simulink model "r2dbe_top"  (R2012b)
settings: Solver=VariableStepDiscrete  SolverMode=SingleTasking  StartTime=0.0  StopTime=10000  RelTol=1e-3
undefined symbols (not defined in the file or in its folder): r2dbe_vdif_lib, sfp, vdif
libraries: xbsIndex_r4 x2792, dspsigops x32, casper_library_delays x29, casper_library_sources x16, casper_library_misc x12, r2dbe_adc_lib x5, xps_library x4, simulink x2
(part 1 of 28)
settings Model: Creator=rprimian  LastModifiedBy=ayoung
settings DataIOCC: SignalLoggingSaveFormat=ModelDataLogs
settings OptimizationCC: InlineParams=on
settings DebuggingCC: SolverPrmCheckMsg=none  FcnCallInpInsideContextMsg=UseLocalSettings  StrictBusMsg=Warning
settings GRTTargetCC: CombineOutputUpdateFcns=off  GRTInterface=on

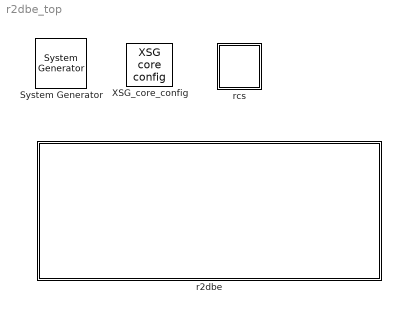
== system r2dbe_top ==
  " System Generator" : xbsIndex_r4/ System Generator  Tag=genX  xilinxfamily=virtex6  part=xc6vsx475t  speed=-1  package=ff1759  synthesis_tool=XST  clock_wrapper=Clock Enables  directory=./r2dbe_top/sysgen  proj_type=Project Navigator  Synth_file=XST Defaults  Impl_file=ISE Defaults  testbench=off  simulink_period=1  sysclk_period=3.9062  dcm_input_clock_period=100  incr_netlist=off  trim_vbits=Everywhere in SubSystem  dbl_ovrd=According to Block Masks  core_generation=According to Block Masks  run_coregen=off  deprecated_control=off  eval_field=0  block_type=sysgen
      settings: block_version=11.4
  XSG_core_config : xps_library/XSG core config  Tag=xps:xsg  hw_sys=ROACH2:sx475t  clk_src=adc0_clk  ROACH_clk_src=dac1_clk  ROACH2_clk_src=adc0_clk  MKDIG_clk_src=sys_clk  clk_rate=256.0  sample_period=1  synthesis_tool=XST
  r2dbe : Subsystem
  rcs : Subsystem  AncestorBlock=casper_library_misc/rcs  mask(rcs){app_src=timestamp, lib_src=git, user_val=2704}
      mask prompts: app_src "Application revision info to capture"; lib_src "CASPER libraries revision info to capture"; user_val "User specified value"
      mask help:
      | Embeds revision control information for the user design and libraries.
      | On failure to locate specified revision information, falls back to
      | timestamps (current time for libraries).
      | A user specified value is also stored.
      mask init:
      | rcs_init(gcb, ...
      |     'app_src', app_src, ...
      |     'lib_src', lib_src);
      mask TypeOptions app_src: timestamp | git | svn
      mask TypeOptions lib_src: timestamp | git | svn

== system r2dbe_top/r2dbe ==
  1PPS : DiscretePulseGenerator  Period=10
  IF0 Band : simulink/Sources/Band-Limited White Noise  Cov=[0.1]  Ts=1  seed=[23341]
  IF1 Band : simulink/Sources/Band-Limited White Noise  Cov=[0.1]  Ts=1  seed=[23341]
  data_mux_0 : Subsystem  mask(r2dbe_data_mux){mux_latency=1, pipeline_delay=1}
      mask prompts: mux_latency "Mux latency:"; pipeline_delay "Output pipeline delay:"
      mask help: Sub-system for mux parameters of the R2DBE.
      mask Display:
      | plot([0 45 45 0 0 ],[0 14.8571 89.1429 104 0 ]);
      | 
      | color('black');port_label('input',1,'sync_in');
      | color('black');port_label('input',2,'adc');
      | color('black');port_label('input',3,'noise');
      | color('black');port_label('input',4,'tone');
      | 
      | color('black');port_label('output',1,'sync');
      | color('black');port_label('output',2,'out');
      | 
      | color('black');disp('\bf{}','texmode','on');
  data_mux_1 : Subsystem  mask(r2dbe_data_mux){mux_latency=1, pipeline_delay=1}
      mask prompts: mux_latency "Mux latency:"; pipeline_delay "Output pipeline delay:"
      mask help: Sub-system for mux parameters of the R2DBE.
      mask Display:
      | plot([0 45 45 0 0 ],[0 14.8571 89.1429 104 0 ]);
      | 
      | color('black');port_label('input',1,'sync_in');
      | color('black');port_label('input',2,'adc');
      | color('black');port_label('input',3,'noise');
      | color('black');port_label('input',4,'tone');
      | 
      | color('black');port_label('output',1,'sync');
      | color('black');port_label('output',2,'out');
      | 
      | color('black');disp('\bf{}','texmode','on');
  delay_0 : Subsystem  mask(r2dbe_delay){max_delay=256, bram_latency=4, pipeline_delay=3}
      mask prompts: max_delay "Max Delay (samples):"; bram_latency "BRAM Latency:"; pipeline_delay "Output pipeline delay:"
      mask help: Sub-system for delay parameters of the R2DBE.
  delay_1 : Subsystem  mask(r2dbe_delay){max_delay=256, bram_latency=4, pipeline_delay=3}
      mask prompts: max_delay "Max Delay (samples):"; bram_latency "BRAM Latency:"; pipeline_delay "Output pipeline delay:"
      mask help: Sub-system for delay parameters of the R2DBE.
  noise_gen_0 : Subsystem  AncestorBlock=r2dbe_adc_lib/noise_gen  mask(r2dbe_noise_gen){}
      mask help: Sub-system for noise generation of the R2DBE.
  noise_gen_1 : Subsystem  AncestorBlock=r2dbe_adc_lib/noise_gen  mask(r2dbe_noise_gen){}
      mask help: Sub-system for noise generation of the R2DBE.
  onepps : Subsystem  AncestorBlock=r2dbe_adc_lib/onepps  mask(r2dbe_onepps){clk_rate=4096 / 16}
      mask prompts: clk_rate "FPGA clock rate (MHz):"
      mask help: Sub-system for 1pps parameters of the R2DBE.
  quantize_0 : r2dbe_adc_lib/quantize  mult_delay=3  add_delay=2  convert_delay=1  pipeline_delay=1  io_delay=3
      link override thresh/io_delay: latency=0  reg_retiming=on
      link override thresh/r2dbe_top_r2dbe_quantize_0_thresh_user_data_out: arith_type=Unsigned  n_bits=32  bin_pt=0  period=1
      link override thresh/reint1: force_arith_type=on  arith_type=Unsigned  force_bin_pt=on  bin_pt=0
      link override thresh/slice_gain: nbits=32  boolean_output=off  mode=Lower Bit Location + Width  bit0=0
  quantize_1 : r2dbe_adc_lib/quantize  mult_delay=3  add_delay=2  convert_delay=1  pipeline_delay=1  io_delay=3
      link override thresh/io_delay: latency=0  reg_retiming=on
      link override thresh/r2dbe_top_r2dbe_quantize_1_thresh_user_data_out: arith_type=Unsigned  n_bits=32  bin_pt=0  period=1
      link override thresh/reint1: force_arith_type=on  arith_type=Unsigned  force_bin_pt=on  bin_pt=0
      link override thresh/slice_gain: nbits=32  boolean_output=off  mode=Lower Bit Location + Width  bit0=0
  snap_2bit_0 : Subsystem  mask(r2dbe_snap){nsamples=14, data_width=32, io_delay=6}
      mask prompts: nsamples "Number of samples (2^?):"; data_width "Data width (bits):"; io_delay "I/O delay:"
      mask help: Sub-system for snapshot parameters of the R2DBE.
      mask init:
      | set_param([gcb, '/data'], 'data_width', data_width);
      mask TypeOptions data_width: 8 | 16 | 32 | 64 | 128
  snap_2bit_1 : Subsystem  mask(r2dbe_snap){nsamples=14, data_width=32, io_delay=6}
      mask prompts: nsamples "Number of samples (2^?):"; data_width "Data width (bits):"; io_delay "I/O delay:"
      mask help: Sub-system for snapshot parameters of the R2DBE.
      mask init:
      | set_param([gcb, '/data'], 'data_width', data_width);
      mask TypeOptions data_width: 8 | 16 | 32 | 64 | 128
  snap_8bit_0 : Subsystem  mask(r2dbe_snap){nsamples=14, data_width=128, io_delay=6}
      mask prompts: nsamples "Number of samples (2^?):"; data_width "Data width (bits):"; io_delay "I/O delay:"
      mask help: Sub-system for snapshot parameters of the R2DBE.
      mask init:
      | set_param([gcb, '/data'], 'data_width', data_width);
      mask TypeOptions data_width: 8 | 16 | 32 | 64 | 128
  snap_8bit_1 : Subsystem  mask(r2dbe_snap){nsamples=14, data_width=128, io_delay=6}
      mask prompts: nsamples "Number of samples (2^?):"; data_width "Data width (bits):"; io_delay "I/O delay:"
      mask help: Sub-system for snapshot parameters of the R2DBE.
      mask init:
      | set_param([gcb, '/data'], 'data_width', data_width);
      mask TypeOptions data_width: 8 | 16 | 32 | 64 | 128
  tengbe_0 : Subsystem  mask(r2dbe_tengbe){slot=0, port=0}
      mask prompts: slot "Card slot:"
      mask help: Sub-system for 10 GbE parameters of the R2DBE.
      mask init:
      | set_param([gcb, '/core'], 'slot', slot);
      | set_param([gcb, '/core'], 'port_r2_sfpp', port);
      mask TypeOptions slot: 0 | 1
      mask TypeOptions port: 0 | 1 | 2 | 3
  tengbe_1 : Subsystem  mask(r2dbe_tengbe){slot=0, port=1}
      mask prompts: slot "Card slot:"
      mask help: Sub-system for 10 GbE parameters of the R2DBE.
      mask init:
      | set_param([gcb, '/core'], 'slot', slot);
      | set_param([gcb, '/core'], 'port_r2_sfpp', port);
      mask TypeOptions slot: 0 | 1
      mask TypeOptions port: 0 | 1 | 2 | 3
  tone_gen_1 : Subsystem  mask(r2dbe_tone_gen){}
      mask help: Sub-system for tone generation of the R2DBE.
  tone_gen_2 : Subsystem  mask(r2dbe_tone_gen){}
      mask help: Sub-system for tone generation of the R2DBE.
  vdif_0 : Subsystem  AncestorBlock=r2dbe_vdif_lib/vdif  mask(r2dbe_vdif){}
      mask help: Sub-system for VDIF parameters of the R2DBE.
  vdif_1 : Subsystem  AncestorBlock=r2dbe_vdif_lib/vdif  mask(r2dbe_vdif){}
      mask help: Sub-system for VDIF parameters of the R2DBE.
  zdok_0 : Subsystem  mask(r2dbe_zdok){zdok=ZDOK 0, nyquist_bw=2048, pipeline_delay=1}
      mask prompts: zdok "ADC board"; nyquist_bw "Nyquist bandwidth (MHz):"; pipeline_delay "Output pipeline delay:"
      mask help: Sub-system for ADC5g parameters of the R2DBE.
      mask init:
      | set_param([gcb, '/adc'], 'adc_brd', zdok);
      mask TypeOptions zdok: ZDOK 0 | ZDOK 1
  zdok_1 : Subsystem  mask(r2dbe_zdok){zdok=ZDOK 1, nyquist_bw=2048, pipeline_delay=1}
      mask prompts: zdok "ADC board"; nyquist_bw "Nyquist bandwidth (MHz):"; pipeline_delay "Output pipeline delay:"
      mask help: Sub-system for ADC5g parameters of the R2DBE.
      mask init:
      | set_param([gcb, '/adc'], 'adc_brd', zdok);
      mask TypeOptions zdok: ZDOK 0 | ZDOK 1
  wires:
  IF0 Band/1 -> zdok_0/1(analog)
  IF1 Band/1 -> zdok_1/1(analog)
  1PPS/1 -> zdok_1/2(ext_sync), zdok_0/2(ext_sync)
  zdok_0/2(data) -> data_mux_0/2(adc)
  data_mux_0/1(sync_out) -> delay_0/1(sync_in)
  data_mux_0/2(out) -> delay_0/2(data_in)
  noise_gen_0/1(noise) -> data_mux_0/3(noise)
  tone_gen_1/1(tone) -> data_mux_0/4(tone)
  onepps/1(sync) -> data_mux_1/1(sync_in), noise_gen_1/1(sync_in), tone_gen_2/1(sync_in), tone_gen_1/1(sync_in), noise_gen_0/1(sync_in), data_mux_0/1(sync_in)
  zdok_0/1(sync) -> onepps/1(gps)
  zdok_1/1(sync) -> onepps/2(maser)
  delay_0/1(sync) -> snap_8bit_0/1(sync_in), quantize_0/1
  delay_0/2(data) -> snap_8bit_0/2(data_in), quantize_0/2
  quantize_0/1 -> snap_2bit_0/1(sync_in), vdif_0/1(sync)
  quantize_0/2 -> snap_2bit_0/2(data_in), vdif_0/2(data)
  vdif_0/1(tx_data) -> tengbe_0/1(tx_data)
  vdif_0/3(tx_end_of_frame) -> tengbe_0/3(tx_eof)
  vdif_0/2(tx_valid) -> tengbe_0/2(tx_valid)
  zdok_1/2(data) -> data_mux_1/2(adc)
  data_mux_1/1(sync_out) -> delay_1/1(sync_in)
  data_mux_1/2(out) -> delay_1/2(data_in)
  noise_gen_1/1(noise) -> data_mux_1/3(noise)
  tone_gen_2/1(tone) -> data_mux_1/4(tone)
  delay_1/1(sync) -> snap_8bit_1/1(sync_in), quantize_1/1
  delay_1/2(data) -> snap_8bit_1/2(data_in), quantize_1/2
  quantize_1/1 -> vdif_1/1(sync), snap_2bit_1/1(sync_in)
  quantize_1/2 -> vdif_1/2(data), snap_2bit_1/2(data_in)
  vdif_1/1(tx_data) -> tengbe_1/1(tx_data)
  vdif_1/3(tx_end_of_frame) -> tengbe_1/3(tx_eof)
  vdif_1/2(tx_valid) -> tengbe_1/2(tx_valid)

== system r2dbe_top/rcs ==
  note: 0 -> revision info
      | 1 -> timestamp
  note: Last modification
      | in seconds since
      | 01-01-1970
  note: 0 -> git
      | 1 -> svn
  note: 0 -> cleanly in revision control
  note: git -> first 28 bits of commit hash
      | svn -> latest revision number
  note: 0 -> revision info
      | 1 -> timestamp
  note: Compile time
      | in seconds since
      | 01-01-1970
  note: 0 -> git
      | 1 -> svn
  note: 0 -> cleanly in revision control
  note: git -> first 28 bits of commit hash
      | svn -> latest revision number
  Concat : xbsIndex_r4/Concat  num_inputs=2  dbl_ovrd=off  block_type=concat
  Concat1 : xbsIndex_r4/Concat  num_inputs=2  dbl_ovrd=off  block_type=concat
  Mux : xbsIndex_r4/Mux  inputs=2  en=off  latency=0  precision=Full  arith_type=Unsigned  n_bits=16  bin_pt=14  quantization=Truncate  overflow=Wrap  dbl_ovrd=off  block_type=mux
      settings: block_version=11.4
  Mux1 : xbsIndex_r4/Mux  inputs=2  en=off  latency=0  precision=Full  arith_type=Unsigned  n_bits=16  bin_pt=14  quantization=Truncate  overflow=Wrap  dbl_ovrd=off  block_type=mux
      settings: block_version=11.4
  Terminator : Terminator
  Terminator1 : Terminator
  Terminator2 : Terminator
  app : Subsystem  Tag=xps:sw_reg  mask{io_dir=To Processor, arith_type=Unsigned, bitwidth=32, bin_pt=0, sample_period=1, latency=0}
      mask prompts: io_dir "I/O direction"; arith_type "Data Type"; bitwidth "Data bitwidth"; bin_pt "Data binary point"; sample_period "Sample period"
      mask init:
      | gw_name = clear_name(gcb);
      | config.source = str2func('software_register_init');
      | config.toplevel = gcb;
      | xBlock( config, {io_dir, arith_type, bitwidth, bin_pt, ... 
      |     sample_period, gw_name, latency});
      mask TypeOptions io_dir: From Processor | To Processor
      mask TypeOptions arith_type: Unsigned | Signed  (2's comp)
  app_dirty : xbsIndex_r4/Constant  const=1  gui_display_data_type=Fixed-point  arith_type=Unsigned  n_bits=1  bin_pt=0  preci_type=Single  exp_width=8  frac_width=24  explicit_period=on  period=1  equ=P=C  opselect=C  inp2=PCIN>>17  opr=+  inp1=P  carry=CIN  dbl_ovrd=off  block_type=constant
      settings: block_version=11.4
  app_info : xbsIndex_r4/Concat  num_inputs=4  dbl_ovrd=off  block_type=concat
  app_info1 : xbsIndex_r4/Concat  num_inputs=4  dbl_ovrd=off  block_type=concat
  app_rcs_type : xbsIndex_r4/Constant  const=0  gui_display_data_type=Fixed-point  arith_type=Unsigned  n_bits=1  bin_pt=0  preci_type=Single  exp_width=8  frac_width=24  explicit_period=on  period=1  equ=P=C  opselect=C  inp2=PCIN>>17  opr=+  inp1=P  carry=CIN  dbl_ovrd=off  block_type=constant
      settings: block_version=11.4
  app_reserved : xbsIndex_r4/Constant  const=0  gui_display_data_type=Fixed-point  arith_type=Unsigned  n_bits=1  bin_pt=0  preci_type=Single  exp_width=8  frac_width=24  explicit_period=on  period=1  equ=P=C  opselect=C  inp2=PCIN>>17  opr=+  inp1=P  carry=CIN  dbl_ovrd=off  block_type=constant
      settings: block_version=11.4
  app_revision : xbsIndex_r4/Constant  const=0  gui_display_data_type=Fixed-point  arith_type=Unsigned  n_bits=28  bin_pt=0  preci_type=Single  exp_width=8  frac_width=24  explicit_period=on  period=1  equ=P=C  opselect=C  inp2=PCIN>>17  opr=+  inp1=P  carry=CIN  dbl_ovrd=off  block_type=constant
      settings: block_version=11.4
  app_timestamp : xbsIndex_r4/Constant  const=1456161552  gui_display_data_type=Fixed-point  arith_type=Unsigned  n_bits=31  bin_pt=0  preci_type=Single  exp_width=8  frac_width=24  explicit_period=on  period=1  equ=P=C  opselect=C  inp2=PCIN>>17  opr=+  inp1=P  carry=CIN  dbl_ovrd=off  block_type=constant
      settings: block_version=11.4
  app_type : xbsIndex_r4/Constant  const=1  gui_display_data_type=Fixed-point  arith_type=Unsigned  n_bits=1  bin_pt=0  preci_type=Single  exp_width=8  frac_width=24  explicit_period=on  period=1  equ=P=C  opselect=C  inp2=PCIN>>17  opr=+  inp1=P  carry=CIN  dbl_ovrd=off  block_type=constant
      settings: block_version=11.4
  lib : Subsystem  Tag=xps:sw_reg  mask{io_dir=To Processor, arith_type=Unsigned, bitwidth=32, bin_pt=0, sample_period=1, latency=0}
      mask prompts: io_dir "I/O direction"; arith_type "Data Type"; bitwidth "Data bitwidth"; bin_pt "Data binary point"; sample_period "Sample period"
      mask init:
      | gw_name = clear_name(gcb);
      | config.source = str2func('software_register_init');
      | config.toplevel = gcb;
      | xBlock( config, {io_dir, arith_type, bitwidth, bin_pt, ... 
      |     sample_period, gw_name, latency});
      mask TypeOptions io_dir: From Processor | To Processor
      mask TypeOptions arith_type: Unsigned | Signed  (2's comp)
  lib_dirty : xbsIndex_r4/Constant  const=1  gui_display_data_type=Fixed-point  arith_type=Unsigned  n_bits=1  bin_pt=0  preci_type=Single  exp_width=8  frac_width=24  explicit_period=on  period=1  equ=P=C  opselect=C  inp2=PCIN>>17  opr=+  inp1=P  carry=CIN  dbl_ovrd=off  block_type=constant
      settings: block_version=11.4
  lib_rcs_type : xbsIndex_r4/Constant  const=0  gui_display_data_type=Fixed-point  arith_type=Unsigned  n_bits=1  bin_pt=0  preci_type=Single  exp_width=8  frac_width=24  explicit_period=on  period=1  equ=P=C  opselect=C  inp2=PCIN>>17  opr=+  inp1=P  carry=CIN  dbl_ovrd=off  block_type=constant
      settings: block_version=11.4
  lib_reserved : xbsIndex_r4/Constant  const=0  gui_display_data_type=Fixed-point  arith_type=Unsigned  n_bits=1  bin_pt=0  preci_type=Single  exp_width=8  frac_width=24  explicit_period=on  period=1  equ=P=C  opselect=C  inp2=PCIN>>17  opr=+  inp1=P  carry=CIN  dbl_ovrd=off  block_type=constant
      settings: block_version=11.4
  lib_revision : xbsIndex_r4/Constant  const=hex2dec('a288ff3')  gui_display_data_type=Fixed-point  arith_type=Unsigned  n_bits=28  bin_pt=0  preci_type=Single  exp_width=8  frac_width=24  explicit_period=on  period=1  equ=P=C  opselect=C  inp2=PCIN>>17  opr=+  inp1=P  carry=CIN  dbl_ovrd=off  block_type=constant
      settings: block_version=11.4
  lib_timestamp : xbsIndex_r4/Constant  const=1456143949  gui_display_data_type=Fixed-point  arith_type=Unsigned  n_bits=31  bin_pt=0  preci_type=Single  exp_width=8  frac_width=24  explicit_period=on  period=1  equ=P=C  opselect=C  inp2=PCIN>>17  opr=+  inp1=P  carry=CIN  dbl_ovrd=off  block_type=constant
      settings: block_version=11.4
  lib_type : xbsIndex_r4/Constant  const=0  gui_display_data_type=Fixed-point  arith_type=Unsigned  n_bits=1  bin_pt=0  preci_type=Single  exp_width=8  frac_width=24  explicit_period=on  period=1  equ=P=C  opselect=C  inp2=PCIN>>17  opr=+  inp1=P  carry=CIN  dbl_ovrd=off  block_type=constant
      settings: block_version=11.4
  user : Subsystem  Tag=xps:sw_reg  mask{io_dir=To Processor, arith_type=Unsigned, bitwidth=32, bin_pt=0, sample_period=1, latency=0}
      mask prompts: io_dir "I/O direction"; arith_type "Data Type"; bitwidth "Data bitwidth"; bin_pt "Data binary point"; sample_period "Sample period"
      mask init:
      | gw_name = clear_name(gcb);
      | config.source = str2func('software_register_init');
      | config.toplevel = gcb;
      | xBlock( config, {io_dir, arith_type, bitwidth, bin_pt, ... 
      |     sample_period, gw_name, latency});
      mask TypeOptions io_dir: From Processor | To Processor
      mask TypeOptions arith_type: Unsigned | Signed  (2's comp)
  user_val : xbsIndex_r4/Constant  const=user_val  gui_display_data_type=Fixed-point  arith_type=Unsigned  n_bits=32  bin_pt=0  preci_type=Single  exp_width=8  frac_width=24  explicit_period=off  period=1  equ=P=C  opselect=C  inp2=PCIN>>17  opr=+  inp1=P  carry=CIN  dbl_ovrd=off  block_type=constant
      settings: block_version=11.4
  wires:
  app/1(sim_reg_out) -> Terminator/1
  user/1(sim_reg_out) -> Terminator2/1
  user_val/1 -> user/1(reg_out)
  app_rcs_type/1 -> app_info/1
  app_reserved/1 -> app_info/2
  app_dirty/1 -> app_info/3
  app_revision/1 -> app_info/4
  app_type/1 -> Concat/1, Mux/1
  app_info/1 -> Mux/2
  app_timestamp/1 -> Mux/3
  Mux/1 -> Concat/2
  Concat/1 -> app/1(reg_out)
  lib/1(sim_reg_out) -> Terminator1/1
  lib_rcs_type/1 -> app_info1/1
  lib_reserved/1 -> app_info1/2
  lib_dirty/1 -> app_info1/3
  lib_revision/1 -> app_info1/4
  lib_type/1 -> Concat1/1, Mux1/1
  app_info1/1 -> Mux1/2
  lib_timestamp/1 -> Mux1/3
  Mux1/1 -> Concat1/2
  Concat1/1 -> lib/1(reg_out)

== system r2dbe_top/r2dbe/data_mux_0 ==
  sync_in : Inport
  adc : Inport  Port=2
  noise : Inport  Port=3
  tone : Inport  Port=4
  Constant : xbsIndex_r4/Constant  const=0  gui_display_data_type=Fixed-point  arith_type=Unsigned  n_bits=128  bin_pt=0  preci_type=Single  exp_width=8  frac_width=24  explicit_period=on  period=1  equ=P=C  opselect=C  inp2=PCIN>>17  opr=+  inp1=P  carry=CIN  dbl_ovrd=off  block_type=constant
  Constant1 : Constant  Value=0
  Slice : xbsIndex_r4/Slice  nbits=2  boolean_output=off  mode=Lower Bit Location + Width  bit1=0  base1=MSB of Input  bit0=0  base0=LSB of Input  dbl_ovrd=off  block_type=slice
  mux : xbsIndex_r4/Mux  inputs=4  en=off  latency=mux_latency  precision=Full  arith_type=Unsigned  n_bits=16  bin_pt=14  quantization=Truncate  overflow=Wrap  dbl_ovrd=off  block_type=mux
  pipeline : Subsystem  AncestorBlock=casper_library_delays/pipeline  mask(pipeline){latency=pipeline_delay}
      mask help:
      | An explicitly laid-out delay line to avoid mapping to SRL16s
      | for use in pipelining to help achieve timing closure.
      mask init:
      | pipeline_init(gcb,'latency',latency);
      settings: AttributesFormatString=Latency = %<latency>
      mask Display:
      | port_label('input', 1, 'd');
      | port_label('output', 1, 'q');
      | disp(['Z^-', num2str(latency)]);
  sel : Subsystem  Tag=xps:sw_reg  AncestorBlock=xps_library/software register  mask(swreg){mode=one value, io_dir=From Processor, io_delay=0, sample_period=1, names=sel, bitwidths=32, arith_types=0, bin_pts=0, sim_port=on, show_format=off}
      mask prompts: io_dir "I/O direction"; io_delay "I/O delay"; sample_period "Sample period"; names "Name:"; bitwidths "Bitwidth:"; arith_types "Type (ufix=0, fix=1, bool=2):"; bin_pts "Binary pt:"; sim_port "Provide sim input/output?"; show_format "Print format string?"
      mask init:
      | swreg_init(gcb)
      settings: AttributesFormatString=1input
      mask TypeOptions mode: one value | fields of equal size | fields of arbitrary size
      mask Callback mode: swreg_cb(gcb);
      mask TypeOptions io_dir: To Processor | From Processor
      mask Callback io_dir:
      | mask_enables = get_param(gcb, 'MaskEnables');
      | mask_names = get_param(gcb, 'MaskNames');
      | if strcmp(get_param(gcb, 'io_dir'), 'To Processor'),
      |     mask_enables{ismember(mask_names, 'sample_period')} = 'off';
      | else
      |     mask_enables{ismember(mask_names, 'sample_period')} = 'on';
      | end
      | set_param(gcb, 'MaskEnables', mask_enables);
      mask Callback bitwidths:
      | swreg_maskcheck(gcb);
      | % blk = gcb;
      | % mode = get_param(blk, 'mode');
      | % current_widths = eval(get_param(blk, 'bitwidths'));
      | % if (strcmp(mode, 'one value') || strcmp(mode, 'fields of equal size')) && (length(current_widths) > 1),
      | %     error('Only one width may be specified for this mode.');
      | % elseif strcmp(mode, 'fields of arbitrary size')
      | %     current_names = textscan(strtrim(strrep(strrep(get_param(blk, 'names'), ']', ''), '[', '')), '%s');
      | %     current_names = current_names{1};
      | %     numios = length(current_names);
      | %     if length(current_widths) ~= numios,
      | %         error('%d field names specified, but %d widths?', numios, length(current_widths));
      | %     end
      | % end
      | % total_width = 0;
      | % for ctr = 1 : length(current_widths),
      | %     total_width = total_width + current_widths(ctr);
      | % end
      | % if total_width > 32,
      | %     error('Total width must be 32 or less, set to %d.', total_width);
      | % end
      mask Callback arith_types:
      | [numios, ~, ~, ~, current_types] = swreg_maskcheck(gcb);
      | % blk = gcb;
      | % mode = get_param(blk, 'mode');
      | % current_types = eval(get_param(blk, 'arith_types'));
      | % numios = length(current_types);
      | % if (strcmp(mode, 'one value') || strcmp(mode, 'fields of equal size')) && (length(current_types) > 1),
      | %     error('Only one type may be specified for this mode.');
      | % elseif strcmp(mode, 'fields of arbitrary size')
      | %     current_names = textscan(strtrim(strrep(strrep(get_param(blk, 'names'), ']', ''), '[', '')), '%s');
      | %     current_names = current_names{1};
      | %     numios = length(current_names);
      | %     if length(current_types) ~= numios,
      | %         error('%d field names specified, but %d types?', numios, length(current_types));
      | %     end
      | % end
      | problem = 0;
      | for ctr = 1 : numios,
      |     t = current_types(ctr);
      |     if (t < 0) || (t > 2),
      |         problem = t;
      |         ctr = numios + 1;
      |     end
      | end
      | if problem ~= 0,
      |     error('Type cannot be %i, must be 0, 1 or 2.', problem);
      | end
      mask Callback bin_pts:
      | swreg_maskcheck(gcb);
      | % blk = gcb;
      | % mode = get_param(blk, 'mode');
      | % current_bins = eval(get_param(blk, 'bin_pts'));
      | % if (strcmp(mode, 'one value') || strcmp(mode, 'fields of equal size')) && (length(current_bins) > 1),
      | %     error('Only one binary pt may be specified for this mode.');
      | % elseif strcmp(mode, 'fields of arbitrary size')
      | %     current_names = textscan(strtrim(strrep(strrep(get_param(blk, 'names'), ']', ''), '[', '')), '%s');
      | %     current_names = current_names{1};
      | %     numios = length(current_names);
      | %     if length(current_bins) ~= numios,
      | %         error('%d field names specified, but %d binary pts?', numios, length(current_bins));
      | %     end
      | % end
  sync_del : Subsystem  AncestorBlock=casper_library_delays/pipeline  mask(pipeline){latency=mux_latency + pipeline_delay}
      mask help:
      | An explicitly laid-out delay line to avoid mapping to SRL16s
      | for use in pipelining to help achieve timing closure.
      mask init:
      | pipeline_init(gcb,'latency',latency);
      settings: AttributesFormatString=Latency = %<latency>
      mask Display:
      | port_label('input', 1, 'd');
      | port_label('output', 1, 'q');
      | disp(['Z^-', num2str(latency)]);
  sync_out : Outport
  out : Outport  Port=2
  wires:
  mux/1 -> pipeline/1(d)
  pipeline/1(q) -> out/1
  Constant1/1 -> sel/1(sim_1)
  sel/1(in_sel) -> Slice/1
  Constant/1 -> mux/2
  tone/1 -> mux/5
  noise/1 -> mux/4
  adc/1 -> mux/3
  sync_del/1(q) -> sync_out/1
  sync_in/1 -> sync_del/1(d)
  Slice/1 -> mux/1

== system r2dbe_top/r2dbe/data_mux_1 ==
  sync_in : Inport
  adc : Inport  Port=2
  noise : Inport  Port=3
  tone : Inport  Port=4
  Constant : xbsIndex_r4/Constant  const=0  gui_display_data_type=Fixed-point  arith_type=Unsigned  n_bits=128  bin_pt=0  preci_type=Single  exp_width=8  frac_width=24  explicit_period=on  period=1  equ=P=C  opselect=C  inp2=PCIN>>17  opr=+  inp1=P  carry=CIN  dbl_ovrd=off  block_type=constant
  Constant1 : Constant  Value=0
  Slice : xbsIndex_r4/Slice  nbits=2  boolean_output=off  mode=Lower Bit Location + Width  bit1=0  base1=MSB of Input  bit0=0  base0=LSB of Input  dbl_ovrd=off  block_type=slice
  mux : xbsIndex_r4/Mux  inputs=4  en=off  latency=mux_latency  precision=Full  arith_type=Unsigned  n_bits=16  bin_pt=14  quantization=Truncate  overflow=Wrap  dbl_ovrd=off  block_type=mux
  pipeline : Subsystem  AncestorBlock=casper_library_delays/pipeline  mask(pipeline){latency=pipeline_delay}
      mask help:
      | An explicitly laid-out delay line to avoid mapping to SRL16s
      | for use in pipelining to help achieve timing closure.
      mask init:
      | pipeline_init(gcb,'latency',latency);
      settings: AttributesFormatString=Latency = %<latency>
      mask Display:
      | port_label('input', 1, 'd');
      | port_label('output', 1, 'q');
      | disp(['Z^-', num2str(latency)]);
  sel : Subsystem  Tag=xps:sw_reg  AncestorBlock=xps_library/software register  mask(swreg){mode=one value, io_dir=From Processor, io_delay=0, sample_period=1, names=sel, bitwidths=32, arith_types=0, bin_pts=0, sim_port=on, show_format=off}
      mask prompts: io_dir "I/O direction"; io_delay "I/O delay"; sample_period "Sample period"; names "Name:"; bitwidths "Bitwidth:"; arith_types "Type (ufix=0, fix=1, bool=2):"; bin_pts "Binary pt:"; sim_port "Provide sim input/output?"; show_format "Print format string?"
      mask init:
      | swreg_init(gcb)
      settings: AttributesFormatString=1input
      mask TypeOptions mode: one value | fields of equal size | fields of arbitrary size
      mask Callback mode: swreg_cb(gcb);
      mask TypeOptions io_dir: To Processor | From Processor
      mask Callback io_dir:
      | mask_enables = get_param(gcb, 'MaskEnables');
      | mask_names = get_param(gcb, 'MaskNames');
      | if strcmp(get_param(gcb, 'io_dir'), 'To Processor'),
      |     mask_enables{ismember(mask_names, 'sample_period')} = 'off';
      | else
      |     mask_enables{ismember(mask_names, 'sample_period')} = 'on';
      | end
      | set_param(gcb, 'MaskEnables', mask_enables);
      mask Callback bitwidths:
      | swreg_maskcheck(gcb);
      | % blk = gcb;
      | % mode = get_param(blk, 'mode');
      | % current_widths = eval(get_param(blk, 'bitwidths'));
      | % if (strcmp(mode, 'one value') || strcmp(mode, 'fields of equal size')) && (length(current_widths) > 1),
      | %     error('Only one width may be specified for this mode.');
      | % elseif strcmp(mode, 'fields of arbitrary size')
      | %     current_names = textscan(strtrim(strrep(strrep(get_param(blk, 'names'), ']', ''), '[', '')), '%s');
      | %     current_names = current_names{1};
      | %     numios = length(current_names);
      | %     if length(current_widths) ~= numios,
      | %         error('%d field names specified, but %d widths?', numios, length(current_widths));
      | %     end
      | % end
      | % total_width = 0;
      | % for ctr = 1 : length(current_widths),
      | %     total_width = total_width + current_widths(ctr);
      | % end
      | % if total_width > 32,
      | %     error('Total width must be 32 or less, set to %d.', total_width);
      | % end
      mask Callback arith_types:
      | [numios, ~, ~, ~, current_types] = swreg_maskcheck(gcb);
      | % blk = gcb;
      | % mode = get_param(blk, 'mode');
      | % current_types = eval(get_param(blk, 'arith_types'));
      | % numios = length(current_types);
      | % if (strcmp(mode, 'one value') || strcmp(mode, 'fields of equal size')) && (length(current_types) > 1),
      | %     error('Only one type may be specified for this mode.');
      | % elseif strcmp(mode, 'fields of arbitrary size')
      | %     current_names = textscan(strtrim(strrep(strrep(get_param(blk, 'names'), ']', ''), '[', '')), '%s');
      | %     current_names = current_names{1};
      | %     numios = length(current_names);
      | %     if length(current_types) ~= numios,
      | %         error('%d field names specified, but %d types?', numios, length(current_types));
      | %     end
      | % end
      | problem = 0;
      | for ctr = 1 : numios,
      |     t = current_types(ctr);
      |     if (t < 0) || (t > 2),
      |         problem = t;
      |         ctr = numios + 1;
      |     end
      | end
      | if problem ~= 0,
      |     error('Type cannot be %i, must be 0, 1 or 2.', problem);
      | end
      mask Callback bin_pts:
      | swreg_maskcheck(gcb);
      | % blk = gcb;
      | % mode = get_param(blk, 'mode');
      | % current_bins = eval(get_param(blk, 'bin_pts'));
      | % if (strcmp(mode, 'one value') || strcmp(mode, 'fields of equal size')) && (length(current_bins) > 1),
      | %     error('Only one binary pt may be specified for this mode.');
      | % elseif strcmp(mode, 'fields of arbitrary size')
      | %     current_names = textscan(strtrim(strrep(strrep(get_param(blk, 'names'), ']', ''), '[', '')), '%s');
      | %     current_names = current_names{1};
      | %     numios = length(current_names);
      | %     if length(current_bins) ~= numios,
      | %         error('%d field names specified, but %d binary pts?', numios, length(current_bins));
      | %     end
      | % end
  sync_del : Subsystem  AncestorBlock=casper_library_delays/pipeline  mask(pipeline){latency=mux_latency + pipeline_delay}
      mask help:
      | An explicitly laid-out delay line to avoid mapping to SRL16s
      | for use in pipelining to help achieve timing closure.
      mask init:
      | pipeline_init(gcb,'latency',latency);
      settings: AttributesFormatString=Latency = %<latency>
      mask Display:
      | port_label('input', 1, 'd');
      | port_label('output', 1, 'q');
      | disp(['Z^-', num2str(latency)]);
  sync_out : Outport
  out : Outport  Port=2
  wires:
  Slice/1 -> mux/1
  sync_in/1 -> sync_del/1(d)
  sync_del/1(q) -> sync_out/1
  adc/1 -> mux/3
  noise/1 -> mux/4
  tone/1 -> mux/5
  Constant/1 -> mux/2
  sel/1(in_sel) -> Slice/1
  Constant1/1 -> sel/1(sim_1)
  pipeline/1(q) -> out/1
  mux/1 -> pipeline/1(d)

== system r2dbe_top/r2dbe/delay_0 ==
  sync_in : Inport
  data_in : Inport  Port=2
  Constant : xbsIndex_r4/Constant  const=1  gui_display_data_type=Boolean  arith_type=Boolean  n_bits=16  bin_pt=14  preci_type=Single  exp_width=8  frac_width=24  explicit_period=on  period=1  equ=P=C  opselect=C  inp2=PCIN>>17  opr=+  inp1=P  carry=CIN  dbl_ovrd=off  block_type=constant
  Constant1 : Constant  Value=0
  bus : Subsystem  AncestorBlock=casper_library_flow_control/bus_create  mask(bus_create){inputNum=16}
      mask prompts: inputNum "Number of inputs:"
      mask init:
      | bus_create_init(gcb,...
      |     'inputNum', inputNum);
  delay_prog : Subsystem  AncestorBlock=casper_library_delays/delay_wideband_prog  mask(delay_wideband_prog){max_delay=max_delay, n_inputs_bits=4, bram_latency=bram_latency, bram_type=Dual Port, async=off}
      mask prompts: max_delay "Max Delay (Sample Clks)"; n_inputs_bits "Number of Simultaneous Inputs(2^?)"; bram_latency "BRAM Latency"; bram_type "Select type of BRAM"; async "asynchronous operation"
      mask init:
      | delay_wideband_prog_init(gcb,...
      |     'max_delay',max_delay,...
      |     'n_inputs_bits',n_inputs_bits,...
      |     'bram_latency',bram_latency,...
      |     'bram_type',bram_type, ...
      |     'async', async);
      mask TypeOptions bram_type: Single Port | Dual Port
  pipeline : Subsystem  AncestorBlock=casper_library_delays/pipeline  mask(pipeline){latency=pipeline_delay}
      mask help:
      | An explicitly laid-out delay line to avoid mapping to SRL16s
      | for use in pipelining to help achieve timing closure.
      mask init:
      | pipeline_init(gcb,'latency',latency);
      settings: AttributesFormatString=Latency = %<latency>
      mask Display:
      | port_label('input', 1, 'd');
      | port_label('output', 1, 'q');
      | disp(['Z^-', num2str(latency)]);
  samples : Subsystem  Tag=xps:sw_reg  AncestorBlock=xps_library/software register  mask(swreg){mode=one value, io_dir=From Processor, io_delay=0, sample_period=1, names=delay, bitwidths=8, arith_types=0, bin_pts=0, sim_port=on, show_format=off}
      mask prompts: io_dir "I/O direction"; io_delay "I/O delay"; sample_period "Sample period"; names "Name:"; bitwidths "Bitwidth:"; arith_types "Type (ufix=0, fix=1, bool=2):"; bin_pts "Binary pt:"; sim_port "Provide sim input/output?"; show_format "Print format string?"
      mask init:
      | swreg_init(gcb)
      settings: AttributesFormatString=1input
      mask TypeOptions mode: one value | fields of equal size | fields of arbitrary size
      mask Callback mode: swreg_cb(gcb);
      mask TypeOptions io_dir: To Processor | From Processor
      mask Callback io_dir:
      | mask_enables = get_param(gcb, 'MaskEnables');
      | mask_names = get_param(gcb, 'MaskNames');
      | if strcmp(get_param(gcb, 'io_dir'), 'To Processor'),
      |     mask_enables{ismember(mask_names, 'sample_period')} = 'off';
      | else
      |     mask_enables{ismember(mask_names, 'sample_period')} = 'on';
      | end
      | set_param(gcb, 'MaskEnables', mask_enables);
      mask Callback bitwidths:
      | swreg_maskcheck(gcb);
      | % blk = gcb;
      | % mode = get_param(blk, 'mode');
      | % current_widths = eval(get_param(blk, 'bitwidths'));
      | % if (strcmp(mode, 'one value') || strcmp(mode, 'fields of equal size')) && (length(current_widths) > 1),
      | %     error('Only one width may be specified for this mode.');
      | % elseif strcmp(mode, 'fields of arbitrary size')
      | %     current_names = textscan(strtrim(strrep(strrep(get_param(blk, 'names'), ']', ''), '[', '')), '%s');
      | %     current_names = current_names{1};
      | %     numios = length(current_names);
      | %     if length(current_widths) ~= numios,
      | %         error('%d field names specified, but %d widths?', numios, length(current_widths));
      | %     end
      | % end
      | % total_width = 0;
      | % for ctr = 1 : length(current_widths),
      | %     total_width = total_width + current_widths(ctr);
      | % end
      | % if total_width > 32,
      | %     error('Total width must be 32 or less, set to %d.', total_width);
      | % end
      mask Callback arith_types:
      | [numios, ~, ~, ~, current_types] = swreg_maskcheck(gcb);
      | % blk = gcb;
      | % mode = get_param(blk, 'mode');
      | % current_types = eval(get_param(blk, 'arith_types'));
      | % numios = length(current_types);
      | % if (strcmp(mode, 'one value') || strcmp(mode, 'fields of equal size')) && (length(current_types) > 1),
      | %     error('Only one type may be specified for this mode.');
      | % elseif strcmp(mode, 'fields of arbitrary size')
      | %     current_names = textscan(strtrim(strrep(strrep(get_param(blk, 'names'), ']', ''), '[', '')), '%s');
      | %     current_names = current_names{1};
      | %     numios = length(current_names);
      | %     if length(current_types) ~= numios,
      | %         error('%d field names specified, but %d types?', numios, length(current_types));
      | %     end
      | % end
      | problem = 0;
      | for ctr = 1 : numios,
      |     t = current_types(ctr);
      |     if (t < 0) || (t > 2),
      |         problem = t;
      |         ctr = numios + 1;
      |     end
      | end
      | if problem ~= 0,
      |     error('Type cannot be %i, must be 0, 1 or 2.', problem);
      | end
      mask Callback bin_pts:
      | swreg_maskcheck(gcb);
      | % blk = gcb;
      | % mode = get_param(blk, 'mode');
      | % current_bins = eval(get_param(blk, 'bin_pts'));
      | % if (strcmp(mode, 'one value') || strcmp(mode, 'fields of equal size')) && (length(current_bins) > 1),
      | %     error('Only one binary pt may be specified for this mode.');
      | % elseif strcmp(mode, 'fields of arbitrary size')
      | %     current_names = textscan(strtrim(strrep(strrep(get_param(blk, 'names'), ']', ''), '[', '')), '%s');
      | %     current_names = current_names{1};
      | %     numios = length(current_names);
      | %     if length(current_bins) ~= numios,
      | %         error('%d field names specified, but %d binary pts?', numios, length(current_bins));
      | %     end
      | % end
  unbus : Subsystem  AncestorBlock=casper_library_flow_control/bus_expand  mask(bus_expand){mode=divisions of equal size, outputNum=16, outputWidth=8, outputBinaryPt=0, outputArithmeticType=0, show_format=off, outputToWorkspace=off, variablePrefix=out, outputToModelAsWell=on}
      mask prompts: outputNum "Number of outputs:"; outputWidth "Output width:"; outputBinaryPt "Output binary point position:"; outputArithmeticType "Output arithmetic type (ufix=0, fix=1, bool=2):"; show_format "Print format string?"; outputToWorkspace "Output to workspace?"; variablePrefix "Variable name prefix:"; outputToModelAsWell "Output to model as well?"
      mask help:
      | Expands a 'bus' made using a bus_create or Xilinx
      | concat block.
      | The input will be divided into the specified number
      | of outputs with the specified arithmetic types.
      | Divisions are made from most significant bit.
      mask init:
      | bus_expand_init(gcb,...
      |     'mode', mode, ...
      |     'outputNum', outputNum, ...
      |     'outputWidth', outputWidth, ...
      |     'outputBinaryPt', outputBinaryPt, ...
      |     'outputArithmeticType', outputArithmeticType, ...
      |     'show_format', show_format, ...
      |     'outputToWorkspace', outputToWorkspace, ...
      |     'variablePrefix', variablePrefix, ...
      |     'outputToModelAsWell', outputToModelAsWell);
      settings: AttributesFormatString=16 outputs
      mask TypeOptions mode: divisions of equal size | divisions of arbitrary size
      mask Callback mode: bus_expand_callback();
      mask Callback outputWidth: bus_expand_callback();
      mask Callback outputToWorkspace: bus_expand_callback();
  sync : Outport
  data : Outport  Port=2
  wires:
  bus/1(bus_out) -> pipeline/1(d)
  pipeline/1(q) -> data/1
  delay_prog/1(sync_out) -> sync/1
  sync_in/1 -> delay_prog/1(sync)
  samples/1(in_delay) -> delay_prog/2(delay)
  unbus/15(out2) -> delay_prog/18(data_in14)
  unbus/16(lsb_out1) -> delay_prog/19(data_in15)
  unbus/1(msb_out16) -> delay_prog/4(data_in0)
  unbus/2(out15) -> delay_prog/5(data_in1)
  unbus/3(out14) -> delay_prog/6(data_in2)
  unbus/4(out13) -> delay_prog/7(data_in3)
  unbus/5(out12) -> delay_prog/8(data_in4)
  unbus/6(out11) -> delay_prog/9(data_in5)
  unbus/7(out10) -> delay_prog/10(data_in6)
  unbus/8(out9) -> delay_prog/11(data_in7)
  unbus/9(out8) -> delay_prog/12(data_in8)
  unbus/10(out7) -> delay_prog/13(data_in9)
  unbus/11(out6) -> delay_prog/14(data_in10)
  unbus/12(out5) -> delay_prog/15(data_in11)
  unbus/13(out4) -> delay_prog/16(data_in12)
  unbus/14(out3) -> delay_prog/17(data_in13)
  data_in/1 -> unbus/1(bus_in)
  delay_prog/16(data_out14) -> bus/15(in15)
  delay_prog/15(data_out13) -> bus/14(in14)
  delay_prog/12(data_out10) -> bus/11(in11)
  delay_prog/17(data_out15) -> bus/16(in16)
  delay_prog/2(data_out0) -> bus/1(in1)
  delay_prog/3(data_out1) -> bus/2(in2)
  delay_prog/4(data_out2) -> bus/3(in3)
  delay_prog/5(data_out3) -> bus/4(in4)
  delay_prog/6(data_out4) -> bus/5(in5)
  delay_prog/7(data_out5) -> bus/6(in6)
  delay_prog/8(data_out6) -> bus/7(in7)
  delay_prog/9(data_out7) -> bus/8(in8)
  delay_prog/10(data_out8) -> bus/9(in9)
  delay_prog/11(data_out9) -> bus/10(in10)
  delay_prog/14(data_out12) -> bus/13(in13)
  delay_prog/13(data_out11) -> bus/12(in12)
  Constant/1 -> delay_prog/3(ld_delay)
  Constant1/1 -> samples/1(sim_1)
